simulink model "wind_with_p_o"  (R2024a)
settings: Solver=VariableStepAuto  StartTime=0  StopTime=40  FixedStep=10e-6  RelTol=1e-3
libraries: spsWindTurbineLib x1, spsPermanentMagnetSynchronousMachineLib x1, spsThreePhaseParallelRLCLoadLib x1, spsThreePhaseVIMeasurementLib x1, sps_lib x1
settings Model: Creator=cbhende  LastModifiedBy=suchi
settings SolverCC: ZeroCrossControl=DisableAll  AlgebraicLoopSolver=TrustRegion
settings DataIOCC: LimitDataPoints=on  SaveFormat=StructureWithTime  SignalLoggingSaveFormat=ModelDataLogs  SaveOutput=off  SignalLogging=off  SaveTime=off  ReturnWorkspaceOutputs=off
settings OptimizationCC: DefaultParameterBehavior=Inlined  ExpressionDepthLimit=2147483647  InitFltsAndDblsToZero=on  EfficientFloat2IntCast=on  LifeSpan=inf
settings DebuggingCC: UnderspecifiedInitializationDetection=Classic  MergeDetectMultiDrivingBlocksExec=none  SolverPrmCheckMsg=warning  FcnCallInpInsideContextMsg=warning  UnconnectedInputMsg=warning  UnconnectedOutputMsg=warning  UnconnectedLineMsg=warning  StateNameClashWarn=warning  SFUnexpectedBacktrackingDiag=warning  SFNoUnconditionalDefaultTransitionDiag=warning  SFExecutionAtInitializationDiag=none  ArithmeticOperatorsInVariantConditions=warning
settings HardwareCC: ProdBitPerPointer=32  ProdBitPerSizeT=32  ProdBitPerPtrDiffT=32  ProdLargestAtomicFloat=None  ProdIntDivRoundTo=Undefined  ProdEndianess=Unspecified  ProdWordSize=32  ProdHWDeviceType=32-bit Generic
settings ModelReferenceCC: PropagateSignalLabelsOutOfModel=off
settings SFSimCC: SimUseLocalCustomCode=off  CustomCodeUndefinedFunction=UseInterfaceOnly
settings RTWCC: RTWUseLocalCustomCode=off  GPUComputeCapability=3.5
settings CodeAppCC: StateflowObjectComments=on
settings GRTTargetCC: TargetLangStandard=C89/C90 (ANSI)  CombineOutputUpdateFcns=off  GRTInterface=on
settings ConfigComp: CovMetricSettings=dw  CovSaveCumulativeToWorkspaceVar=on  CovSaveSingleToWorkspaceVar=on  CovExternalEMLEnable=off
settings SimscapeCC: SimscapeNormalizeSystem=off

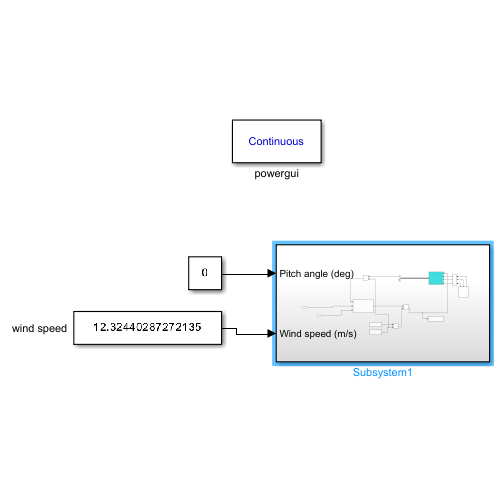
[thumbnail: Simulink's stored preview of the top-level diagram]
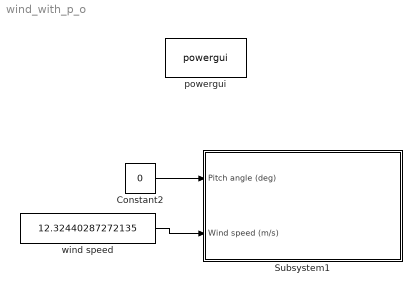
== system wind_with_p_o ==
  Constant2 : Constant  Value=0
  Subsystem1 : Subsystem
  powergui : sps_lib/powergui  Priority=1  SimulationMode=Continuous  SampleTime=1e-5  frequency=60  Iterations=50  frequencyindice=0  Pbase=100e6  ErrMax=1e-4  UnitsV=kV  UnitsW=MW  buscounter=0  FunctionMessages=off  echomessages=off  EnableUseOfTLC=off  CurrentSourceSwitches=off  DisableSnubberDevices=off  DisableRonSwitches=off  DisableVfSwitches=off  DisplayEquations=off  AutomaticDiscreteSolvers=off  SolverType=Tustin/Backward Euler (TBE)  Interpol=off  ExternalGateDelay=off  methode=off  Ts=100  x0status=blocks  SPID=on  SwTol=0  HookPort=off  NonlinearTolerance=1e-4  nMaxIteration=100  ContinueOnMaxIteration=off  RestoreLinks=warning  ResistiveCurrentMeasurement=off  Frange=[0:2:500]  Ylog=off  Xlog=on  ShowGrid=off  save=off  variable=ZData  structure=0  ZoomFFT=off  StartTime=0.0  cycles=1  DisplayStyle=1  fundamental=60  FreqAxis=off  MaxFrequency=1000  frequencyindicesteady=1  RmsSteady=1  display=off
  wind speed : Constant  Value=12.32440287272135
  wires:
  Constant2/1 -> Subsystem1/1(Pitch angle (deg))
  wind speed/1 -> Subsystem1/2(Wind speed (m/s))

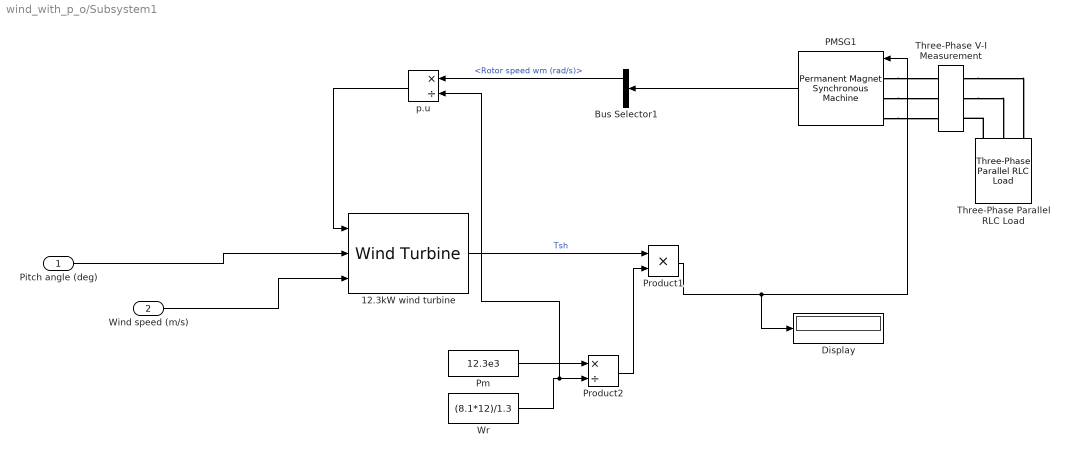
== system wind_with_p_o/Subsystem1 ==
  Pitch angle (deg) : Inport
  Wind speed (m/s) : Inport  Port=2
  "12.3kW wind turbine " : spsWindTurbineLib/Wind Turbine  Pnom=12.3e3  Pelec_base=12.3e3/0.9  wind_base=12  P_wind_base=0.85  speed_nom=1.2  pitch_angle=0  c1_c6="[0.51763          116          0.4            5           21     0.006795]"  cp_nom=0.48  lambda_nom=8.1
  Bus Selector1 : BusSelector  OutputSignals=Rotor speed wm (rad/s),Electromagnetic torque Te (N*m)
  Display : Display
  PMSG1 : spsPermanentMagnetSynchronousMachineLib/Permanent Magnet Synchronous Machine  NbPhases=3  FluxDistribution=Sinusoidal  RotorType=Salient-pole  MechanicalLoad=Torque Tm  PresetModel=No  ShowDetailedParameters=on  MeasurementBus=off  Resistance=0.0485  Inductance=8.5e-3  dqInductances=[0.395e-3 0.395e-3]  La=0.000835  MachineConstant=Flux linkage established by magnets (V.s)  Flux=0.1194  VoltageCst=108.2838  TorqueCst=0.8955  Flat=120  Mechanical=[0.01197 0.001189 5]  PolePairs=5  InitialConditions=[0,0, 0,0]  InitialConditions5ph=[0 0 0 0 0 0]  RefAngle=90 degrees behind phase A axis (modified Park)  IterativeDiscreteModel=Trapezoidal non iterative  TsBlock=-1  TsPowergui=0
  Pm : Constant  Value=12.3e3
  Product1 : Product
  Product2 : Product  Inputs=*/
  Three-Phase Parallel RLC Load : spsThreePhaseParallelRLCLoadLib/Three-Phase Parallel RLC Load  LConnTagsString=A|B|C  Configuration=Y (grounded)  NominalVoltage=400  Vabc=[1e3 1e3 1e3]  Vabcp=[1e3 1e3 1e3]  NominalFrequency=50  UnbalancedPower=off  ActivePower=1e3  InductivePower=1  CapacitivePower=1  Pabc=[10e3 9e3 11e3]  QLabc=[100 90 110]  QCabc=[100 90 110]  Pabcp=[10e3 9e3 11e3]  QLabcp=[100 90 110]  QCabcp=[100 90 110]  Measurements=None  LoadType=constant Z
  Three-Phase V-I Measurement : spsThreePhaseVIMeasurementLib/Three-Phase V-I Measurement  VoltageMeasurement=no  SetLabelV=off  LabelV=Vabc  Vpu=off  VpuLL=off  CurrentMeasurement=no  SetLabelI=off  LabelI=Iabc  Ipu=off  Pbase=100e6  Vbase=500e3  OutputType=Complex  PhasorSimulation=off  PSBequivalent=0
  Wr : Constant  Value=(8.1*12)/1.3
  p.u : Product  Inputs=*/
  wires:
  PMSG1/1 -> Bus Selector1/1
  Wr/1 -> p.u/2, Product2/2
  Bus Selector1/1 -> p.u/1  "<Rotor speed wm (rad/s)>"
  Pm/1 -> Product2/1
  p.u/1 -> "12.3kW wind turbine "/1
  Product1/1 -> PMSG1/1, Display/1
  Product2/1 -> Product1/2
  "12.3kW wind turbine "/1 -> Product1/1  "Tsh"
  Pitch angle (deg)/1 -> "12.3kW wind turbine "/2
  Wind speed (m/s)/1 -> "12.3kW wind turbine "/3
  connections:
  PMSG1/LConn2 -- Three-Phase V-I Measurement/LConn2
  PMSG1/LConn3 -- Three-Phase V-I Measurement/LConn3
  PMSG1/LConn1 -- Three-Phase V-I Measurement/LConn1
  Three-Phase Parallel RLC Load/LConn1 -- Three-Phase V-I Measurement/RConn3
  Three-Phase V-I Measurement/RConn2 -- Three-Phase Parallel RLC Load/LConn2
  Three-Phase V-I Measurement/RConn1 -- Three-Phase Parallel RLC Load/LConn3
